simulink library "adrc_lib"  (R2018a)
settings: Solver=VariableStepAuto  StartTime=0.0  StopTime=10.0  RelTol=1e-3
undefined symbols (not defined in the file): delta, DiscIntNeverNeededParam, DistObs_K1, DistObs_K2, DistObs_K3, TsFast
libraries: ctrl_lib x6, $bdroot x1
settings Model: Creator=uids8840  LastModifiedBy=elrobotista
settings CodeAppCC: StateflowObjectComments=on

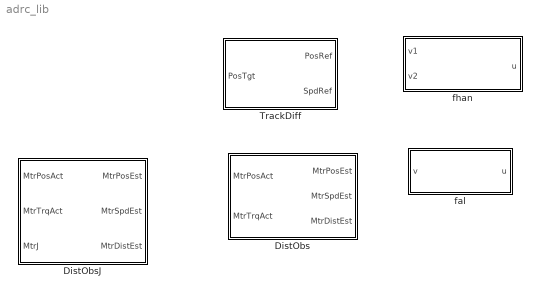
== system adrc_lib ==
  DistObs : Subsystem  SystemSampleTime=1/30e3  mask{ts=1e-3, Jm=1e-6, k1=0, k2=0, k3=0}
      mask prompts: ts "Execution rate [s]"; Jm "Motor Inertia:"; k1 "Gain K1:"; k2 "Gain K2:"; k3 "Gain K3:"
  DistObsJ : Subsystem  SystemSampleTime=1/30e3  mask{ts=TsFast, k1=DistObs_K1, k2=DistObs_K2, k3=DistObs_K3}
      mask prompts: ts "Execution rate [s]"; k1 "Gain K1:"; k2 "Gain K2:"; k3 "Gain K3:"
  TrackDiff : Subsystem  mask{ts=1e-3, h0=1e-3, r0=10e3}
      mask prompts: ts "Exeuction rate [s]:"
  fal : Subsystem  mask{a=0.5, d=1e-3}
      mask prompts: a "Agressivenes [alpha]"; d "Boundary layer [delta]"
  fhan : Subsystem  mask{r0=10e3, h0=1e-3}
      mask prompts: r0 "Agressivenes [r0]"; h0 "Time step [h0]"

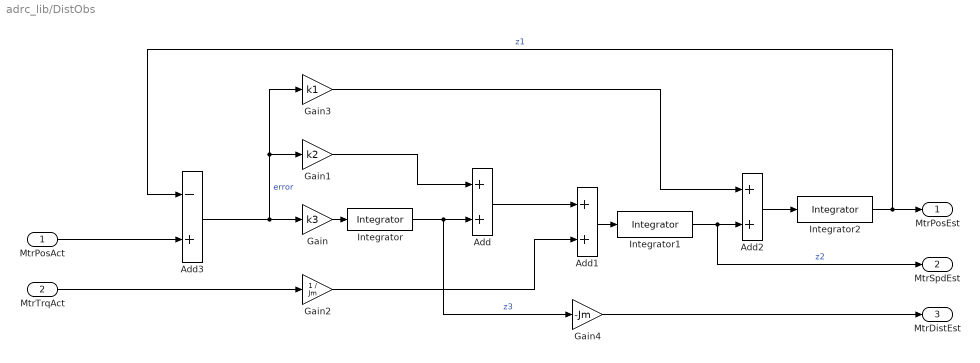
== system adrc_lib/DistObs ==
  MtrPosAct : Inport
  MtrTrqAct : Inport  Port=2
  Add : Sum
  Add1 : Sum
  Add2 : Sum
  Add3 : Sum  Inputs=-+
  Gain : Gain  Gain=k3
      settings: AttributesFormatString=%<Gain>
  Gain1 : Gain  Gain=k2
      settings: AttributesFormatString=%<Gain>
  Gain2 : Gain  Gain=1 / Jm
      settings: AttributesFormatString=%<Gain>
  Gain3 : Gain  Gain=k1
      settings: AttributesFormatString=%<Gain>
  Gain4 : Gain  Gain=-Jm
      settings: AttributesFormatString=%<Gain>
  Integrator : ctrl_lib/Integrator  ts=ts  max_lim=inf  min_lim=-inf
  Integrator1 : ctrl_lib/Integrator  ts=ts  max_lim=inf  min_lim=-inf
  Integrator2 : ctrl_lib/Integrator  ts=ts  max_lim=inf  min_lim=-inf
  MtrPosEst : Outport
  MtrSpdEst : Outport  Port=2
  MtrDistEst : Outport  Port=3
  wires:
  Gain3/1 -> Add2/1
  Add/1 -> Add1/1
  Integrator/1 -> Gain4/1, Add/2  "z3"
  Gain1/1 -> Add/1
  Integrator1/1 -> MtrSpdEst/1, Add2/2  "z2"
  Gain/1 -> Integrator/1
  Integrator2/1 -> MtrPosEst/1, Add3/1  "z1"
  Add2/1 -> Integrator2/1
  MtrPosAct/1 -> Add3/2
  Add1/1 -> Integrator1/1
  Gain2/1 -> Add1/2
  Add3/1 -> Gain3/1, Gain1/1, Gain/1  "error"
  MtrTrqAct/1 -> Gain2/1
  Gain4/1 -> MtrDistEst/1

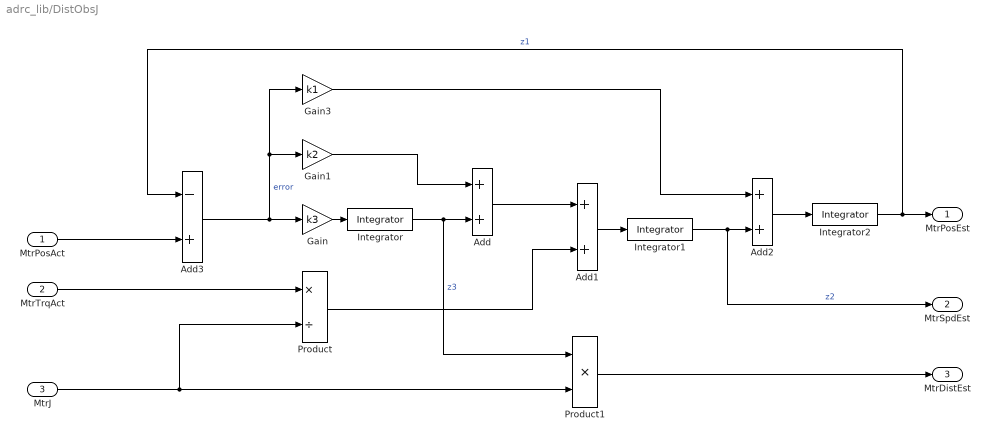
== system adrc_lib/DistObsJ ==
  MtrPosAct : Inport
  MtrTrqAct : Inport  Port=2
  MtrJ : Inport  Port=3
  Add : Sum
  Add1 : Sum
  Add2 : Sum
  Add3 : Sum  Inputs=-+
  Gain : Gain  Gain=k3
      settings: AttributesFormatString=%<Gain>
  Gain1 : Gain  Gain=k2
      settings: AttributesFormatString=%<Gain>
  Gain3 : Gain  Gain=k1
      settings: AttributesFormatString=%<Gain>
  Integrator : ctrl_lib/Integrator  ts=ts  max_lim=1e7  min_lim=-1e7
  Integrator1 : ctrl_lib/Integrator  ts=ts  max_lim=1e7  min_lim=-1e7
  Integrator2 : ctrl_lib/Integrator  ts=ts  max_lim=1e7  min_lim=-1e7
  Product : Product  Inputs=*/
  Product1 : Product  Inputs=**
  MtrPosEst : Outport
  MtrSpdEst : Outport  Port=2
  MtrDistEst : Outport  Port=3
  wires:
  Product1/1 -> MtrDistEst/1
  MtrTrqAct/1 -> Product/1
  Add3/1 -> Gain/1, Gain1/1, Gain3/1  "error"
  Product/1 -> Add1/2
  Add1/1 -> Integrator1/1
  MtrPosAct/1 -> Add3/2
  Add2/1 -> Integrator2/1
  Integrator2/1 -> Add3/1, MtrPosEst/1  "z1"
  Gain/1 -> Integrator/1
  Integrator1/1 -> Add2/2, MtrSpdEst/1  "z2"
  Gain1/1 -> Add/1
  Integrator/1 -> Product1/1, Add/2  "z3"
  Add/1 -> Add1/1
  Gain3/1 -> Add2/1
  MtrJ/1 -> Product/2, Product1/2

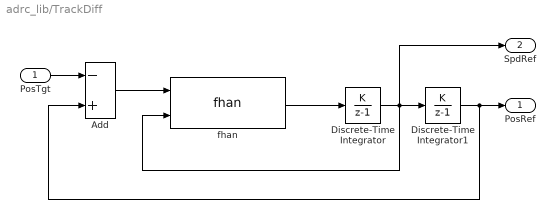
== system adrc_lib/TrackDiff ==
  PosTgt : Inport
  Add : Sum  Inputs=-+
  Discrete-Time Integrator : DiscreteIntegrator  IntegratorMethod=Accumulation: Forward Euler  gainval=ts  SampleTime=-1  ICPrevOutput=DiscIntNeverNeededParam  ICPrevScaledInput=DiscIntNeverNeededParam
  Discrete-Time Integrator1 : DiscreteIntegrator  IntegratorMethod=Accumulation: Forward Euler  gainval=ts  SampleTime=-1  ICPrevOutput=DiscIntNeverNeededParam  ICPrevScaledInput=DiscIntNeverNeededParam
  fhan : $bdroot/fhan  r0=r0  h0=h0
  PosRef : Outport
  SpdRef : Outport  Port=2
  wires:
  PosTgt/1 -> Add/1
  Add/1 -> fhan/1
  fhan/1 -> Discrete-Time Integrator/1
  Discrete-Time Integrator/1 -> SpdRef/1, fhan/2, Discrete-Time Integrator1/1
  Discrete-Time Integrator1/1 -> Add/2, PosRef/1

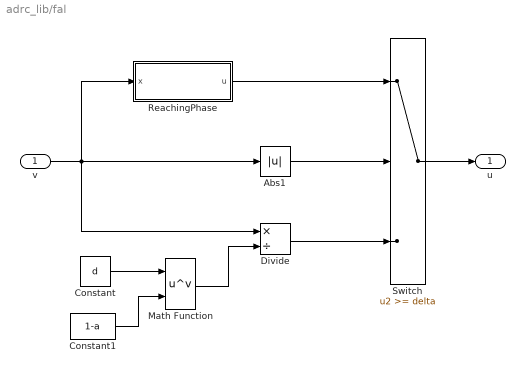
== system adrc_lib/fal ==
  v : Inport
  Abs1 : Abs
  Constant : Constant  Value=d  OutDataTypeStr=single
  Constant1 : Constant  Value=1-a  OutDataTypeStr=single
  Divide : Product  Inputs=*/
  Math Function : Math  Operator=pow  SaturateOnIntegerOverflow=on
  ReachingPhase : Subsystem
  Switch : Switch  Threshold=delta
      settings: AttributesFormatString=%<Criteria>
  u : Outport
  wires:
  v/1 -> ReachingPhase/1(x), Divide/1, Abs1/1
  Divide/1 -> Switch/3
  Constant/1 -> Math Function/1
  Math Function/1 -> Divide/2
  Switch/1 -> u/1
  Abs1/1 -> Switch/2
  Constant1/1 -> Math Function/2
  ReachingPhase/1(u) -> Switch/1

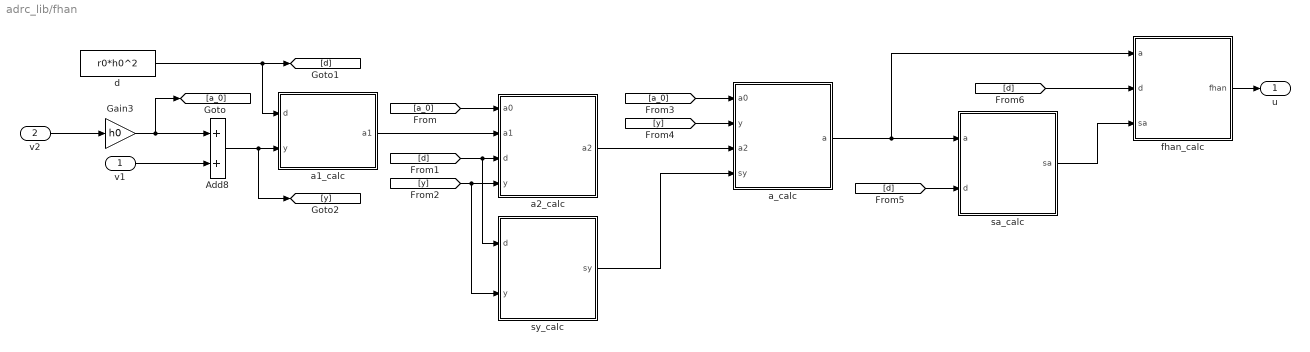
== system adrc_lib/fhan ==
  v1 : Inport
  v2 : Inport  Port=2
  Add8 : Sum
  Gain3 : Gain  Gain=h0
  a1_calc : Subsystem
  a2_calc : Subsystem
  a_calc : Subsystem
  d : Constant  Value=r0*h0^2  OutDataTypeStr=single
  fhan_calc : Subsystem
  sa_calc : Subsystem
  sy_calc : Subsystem
  u : Outport
  wires:
  v1/1 -> Add8/2
  v2/1 -> Gain3/1
  sy_calc/1(sy) -> a_calc/4(sy)
  [d] -> sa_calc/2(d)
  [d] -> a2_calc/3(d), sy_calc/1(d)
  [y] -> a2_calc/4(y), sy_calc/2(y)
  sa_calc/1(sa) -> fhan_calc/3(sa)
  [d] -> fhan_calc/2(d)
  d/1 -> [d], a1_calc/1(d)
  Add8/1 -> a1_calc/2(y), [y]
  Gain3/1 -> [a_0], Add8/1
  fhan_calc/1(fhan) -> u/1
  a_calc/1(a) -> sa_calc/1(a), fhan_calc/1(a)
  [y] -> a_calc/2(y)
  a1_calc/1(a1) -> a2_calc/2(a1)
  [a_0] -> a2_calc/1(a0)
  [a_0] -> a_calc/1(a0)
  a2_calc/1(a2) -> a_calc/3(a2)

== system adrc_lib/fal/ReachingPhase ==
  x : Inport
  Abs : Abs
  Constant : Constant  Value=a  OutDataTypeStr=single
  Math Function1 : Math  Operator=pow  SaturateOnIntegerOverflow=on
  Product : Product  OutDataTypeStr=Inherit: Same as first input
  Sign : Signum
  u : Outport
  wires:
  Product/1 -> u/1
  Math Function1/1 -> Product/1
  Abs/1 -> Math Function1/1
  Sign/1 -> Product/2
  Constant/1 -> Math Function1/2
  x/1 -> Sign/1, Abs/1

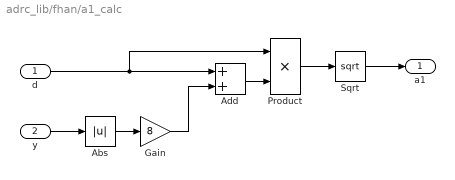
== system adrc_lib/fhan/a1_calc ==
  d : Inport
  y : Inport  Port=2
  Abs : Abs
  Add : Sum
  Gain : Gain  Gain=8
  Product : Product
  Sqrt : Sqrt  SaturateOnIntegerOverflow=on
  a1 : Outport
  wires:
  Sqrt/1 -> a1/1
  Product/1 -> Sqrt/1
  Add/1 -> Product/2
  Gain/1 -> Add/2
  Abs/1 -> Gain/1
  y/1 -> Abs/1
  d/1 -> Add/1, Product/1

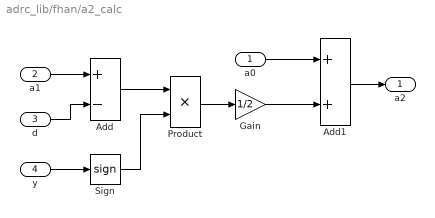
== system adrc_lib/fhan/a2_calc ==
  a0 : Inport
  a1 : Inport  Port=2
  d : Inport  Port=3
  y : Inport  Port=4
  Add : Sum  Inputs=+-
  Add1 : Sum
  Gain : Gain  Gain=1/2
  Product : Product
  Sign : Signum
  a2 : Outport
  wires:
  a0/1 -> Add1/1
  Gain/1 -> Add1/2
  Product/1 -> Gain/1
  Sign/1 -> Product/2
  Add/1 -> Product/1
  y/1 -> Sign/1
  d/1 -> Add/2
  a1/1 -> Add/1
  Add1/1 -> a2/1

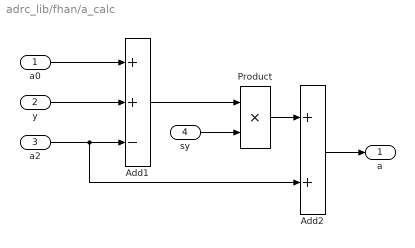
== system adrc_lib/fhan/a_calc ==
  a0 : Inport
  y : Inport  Port=2
  a2 : Inport  Port=3
  sy : Inport  Port=4
  Add1 : Sum  Inputs=++-
  Add2 : Sum
  Product : Product
  a : Outport
  wires:
  Product/1 -> Add2/1
  sy/1 -> Product/2
  Add1/1 -> Product/1
  a2/1 -> Add1/3, Add2/2
  y/1 -> Add1/2
  a0/1 -> Add1/1
  Add2/1 -> a/1

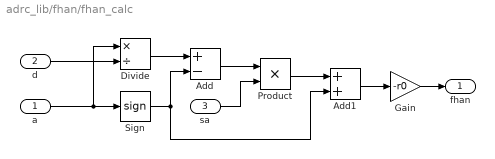
== system adrc_lib/fhan/fhan_calc ==
  a : Inport
  d : Inport  Port=2
  sa : Inport  Port=3
  Add : Sum  Inputs=+-
  Add1 : Sum
  Divide : Product  Inputs=*/
  Gain : Gain  Gain=-r0
  Product : Product
  Sign : Signum
  fhan : Outport
  wires:
  Product/1 -> Add1/1
  Add1/1 -> Gain/1
  sa/1 -> Product/2
  Add/1 -> Product/1
  Sign/1 -> Add/2, Add1/2
  Divide/1 -> Add/1
  a/1 -> Sign/1, Divide/1
  Gain/1 -> fhan/1
  d/1 -> Divide/2

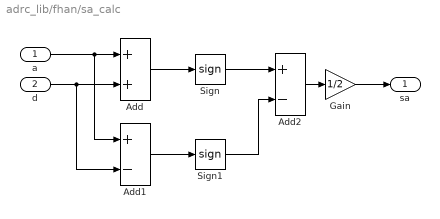
== system adrc_lib/fhan/sa_calc ==
  a : Inport
  d : Inport  Port=2
  Add : Sum
  Add1 : Sum  Inputs=+-
  Add2 : Sum  Inputs=+-
  Gain : Gain  Gain=1/2
  Sign : Signum
  Sign1 : Signum
  sa : Outport
  wires:
  Add2/1 -> Gain/1
  Sign1/1 -> Add2/2
  Sign/1 -> Add2/1
  Add1/1 -> Sign1/1
  Add/1 -> Sign/1
  a/1 -> Add/1, Add1/1
  d/1 -> Add1/2, Add/2
  Gain/1 -> sa/1

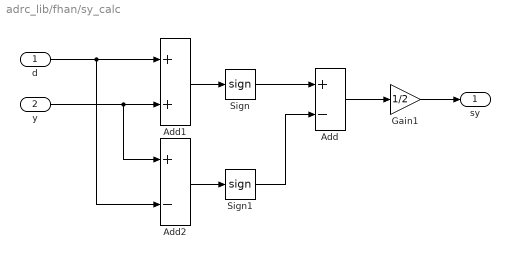
== system adrc_lib/fhan/sy_calc ==
  d : Inport
  y : Inport  Port=2
  Add : Sum  Inputs=+-
  Add1 : Sum
  Add2 : Sum  Inputs=+-
  Gain1 : Gain  Gain=1/2
  Sign : Signum
  Sign1 : Signum
  sy : Outport
  wires:
  Add/1 -> Gain1/1
  Add2/1 -> Sign1/1
  Sign1/1 -> Add/2
  Sign/1 -> Add/1
  Add1/1 -> Sign/1
  Gain1/1 -> sy/1
  d/1 -> Add1/1, Add2/2
  y/1 -> Add1/2, Add2/1
